simulink subsystem "TwoTanks_Sub_Laminar"  (R2023b)
settings: Solver=VariableStepAuto  StartTime=0.0  StopTime=10.0  RelTol=1e-3
libraries: cstblocks x1
settings Model: Creator=HP  LastModifiedBy=HP

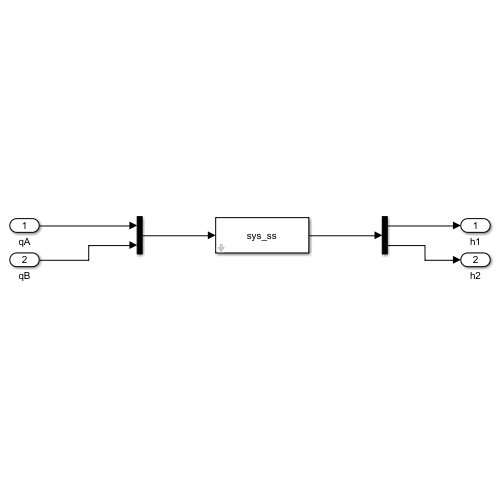
[thumbnail: Simulink's stored preview of the top-level diagram]
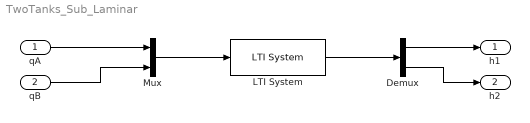
== system TwoTanks_Sub_Laminar ==
  qA : Inport
  qB : Inport  Port=2
  Demux : Demux  Outputs=2
  LTI System : cstblocks/LTI System  sys=sys_ss  IC=h  PadeOrder=0
  Mux : Mux  Inputs=2
  h1 : Outport
  h2 : Outport  Port=2
  wires:
  qA/1 -> Mux/1
  qB/1 -> Mux/2
  Mux/1 -> LTI System/1
  LTI System/1 -> Demux/1
  Demux/1 -> h1/1
  Demux/2 -> h2/1
